simulink model "espesadorReal_1202"  (R2017a)
settings: Solver=VariableStepAuto  StartTime=0.0  StopTime=simTime  RelTol=1e-3  EnableMultiTasking=on
values from neighbouring files (symbols this model uses):
  a1 = 29.6547    [parametrosEmpty.m]
  a2 = 1.8198    [parametrosEmpty.m]
  a3 = 13.2250    (= 13.225)    [parametrosEmpty.m]
  B = 12    [parametrosEmpty.m]
  b0 = -1.3102    [parametrosEmpty.m]
  b1 = 25.8137    [parametrosEmpty.m]
  b2 = 40.3845    [parametrosEmpty.m]
  b3 = 78.1795    [parametrosEmpty.m]
  b4 = 1000    [parametrosEmpty.m]
  c0 = 1.6005e+03    (= 1600.5)    [parametrosEmpty.m]
  c1 = -512.8365    [parametrosEmpty.m]
  Cdata = linspace(0,phi_max,M)    [parametrosEmpty.m]
  Ddata = zeros(size(Cdata))    [parametrosEmpty.m]
  Dt = 1    [parametrosEmpty.m]
  Dz = (B+H)/N    (= 0.0690476190476)    [parametrosEmpty.m]
  jf = ceil(H/Dz)    [parametrosEmpty.m]
  kappa = 220.97    [parametrosEmpty.m]
  L = zeros(2,N+3)    [parametrosEmpty.m]
  lambda = 1./(Dz*A)    [parametrosEmpty.m]
  m = 8.68    [parametrosEmpty.m]
  mu = lambda/Dz    [parametrosEmpty.m]
  N = 210    [parametrosEmpty.m]
  n_rz = 9.65    [parametrosEmpty.m]
  phi0 = zeros(N+3,1)    [parametrosEmpty.m]
  phi_c = 0.2    [parametrosEmpty.m]
  phi_f = weight_to_volume_fraction(0.1,rho_s,rho_f)    [parametrosEmpty.m]
  rho_f = 1000    [parametrosEmpty.m]
  rho_s = 2750    [parametrosEmpty.m]
  theta = 0.2    [parametrosEmpty.m]
  u10 = zeros(N+3,1)    [parametrosEmpty.m]
  u20 = zeros(N+3,1)    [parametrosEmpty.m]
  u30 = zeros(N+3,1)    [parametrosEmpty.m]
  v_max = 25/3600    (= 0.00694444444444)    [parametrosEmpty.m]
  w0 = zeros(N+3,1)    [parametrosEmpty.m]
  y = abs(filter(b,1,SimResults.DV(dv).TimeSeries))    [plotter.m]
  Z = (-(H+Dz):Dz:(B+Dz))'    [parametrosEmpty.m]
undefined symbols (not defined in the file or in its folder): A, Cf_seed, Cf_sigma, Cz, DiscIntNeverNeededParam, p1_seed, p1_sigma, Qf_seed, Qf_sigma, startThickener
settings Model: SimulationMode=rapid-accelerator  ExtModeTrigDuration=100  Creator=pablo  LastModifiedBy=Pablo Diaz
settings DataIOCC: SaveOutput=off  StateSaveName=tmp_raccel_xout  SignalLoggingName=tmp_raccel_logsout
settings OptimizationCC: EfficientMapNaN2IntZero=off  LifeSpan=inf
settings DebuggingCC: SFUnexpectedBacktrackingDiag=warning  SFNoUnconditionalDefaultTransitionDiag=warning  SFExecutionAtInitializationDiag=none
settings HardwareCC: TargetBitPerPointer=64  TargetBitPerSizeT=64  TargetBitPerPtrDiffT=64  TargetLongLongMode=on  TargetIntDivRoundTo=Zero  TargetEndianess=LittleEndian  TargetWordSize=64  TargetHWDeviceType=MATLAB Host  ProdEqTarget=off
settings RTWCC: SystemTargetFile=raccel.tlc  TemplateMakefile=raccel_default_tmf  RTWVerbose=off  RTWUseSimCustomCode=on
settings CodeAppCC: GenerateComments=off  MaxIdLength=128  MangleLength=10  SimulinkBlockComments=off
settings RaccelTargetCC: GeneratePreprocessorConditionals=Use local settings  ERTFirstTimeCompliant=off  MultiInstanceERTCode=off  ENABLE_SLEXEC_SSBRIDGE=0  RTWCAPIParams=on
settings ConfigComp: CovMetricSettings=dw  CovHtmlReporting=on  CovSaveCumulativeToWorkspaceVar=on  CovSaveSingleToWorkspaceVar=on  CovExternalEMLEnable=off

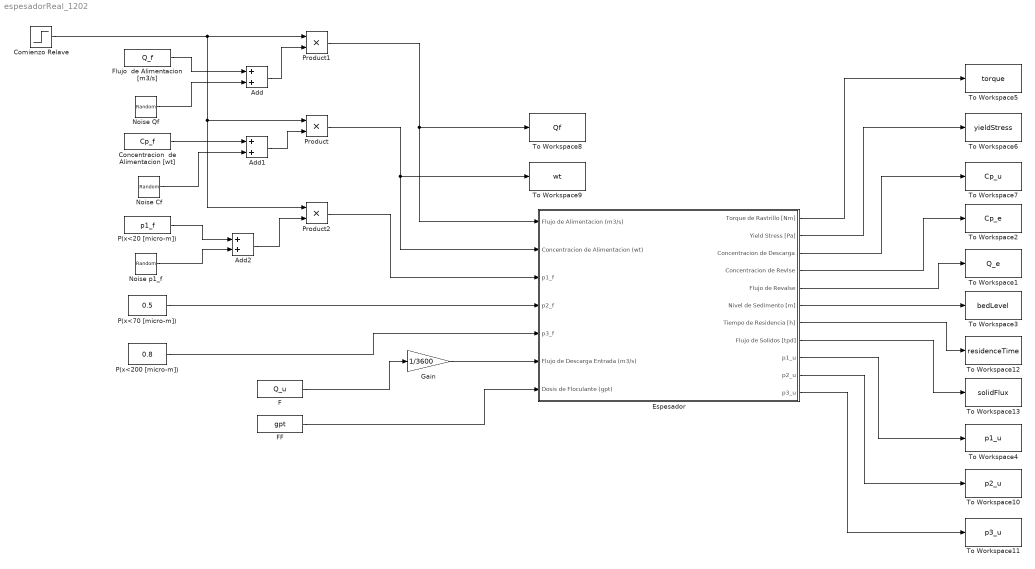
== system espesadorReal_1202 ==
  Add : Sum
  Add1 : Sum
  Add2 : Sum
  Comienzo Relave : Step  Time=startThickener  SampleTime=0
  Concentracion  de Alimentacion [wt] : FromWorkspace  VariableName=Cp_f  SampleTime=0
  Espesador : Subsystem
  F : FromWorkspace  VariableName=Q_u  SampleTime=0
  FF : FromWorkspace  VariableName=gpt  SampleTime=0
  Flujo  de Alimentacion [m3/s] : FromWorkspace  VariableName=Q_f  SampleTime=0
  Gain : Gain  Gain=1/3600
  Noise Cf : RandomNumber  Variance=Cf_sigma^2  Seed=Cf_seed  SampleTime=30*Dt
  Noise Qf : RandomNumber  Variance=Qf_sigma^2  Seed=Qf_seed  SampleTime=30*Dt
  Noise p1_f : RandomNumber  Variance=p1_sigma^2  Seed=p1_seed  SampleTime=30*Dt
  P(x<20 [micro-m]) : FromWorkspace  VariableName=p1_f  SampleTime=0
  P(x<200 [micro-m]) : Constant  Value=0.8
  P(x<70 [micro-m]) : Constant  Value=0.5
  Product : Product
  Product1 : Product
  Product2 : Product
  To Workspace1 : ToWorkspace  VariableName=Q_e  SaveFormat=Structure With Time  SampleTime=-1
  To Workspace10 : ToWorkspace  VariableName=p2_u  SaveFormat=Structure With Time  SampleTime=-1
  To Workspace11 : ToWorkspace  VariableName=p3_u  SaveFormat=Structure With Time  SampleTime=-1
  To Workspace12 : ToWorkspace  VariableName=residenceTime  SaveFormat=Structure With Time  SampleTime=-1
  To Workspace13 : ToWorkspace  VariableName=solidFlux  SaveFormat=Structure With Time  SampleTime=-1
  To Workspace2 : ToWorkspace  VariableName=Cp_e  SaveFormat=Structure With Time  SampleTime=-1
  To Workspace3 : ToWorkspace  VariableName=bedLevel  SaveFormat=Structure With Time  SampleTime=-1
  To Workspace4 : ToWorkspace  VariableName=p1_u  SaveFormat=Structure With Time  SampleTime=-1
  To Workspace5 : ToWorkspace  VariableName=torque  SaveFormat=Structure With Time  SampleTime=-1
  To Workspace6 : ToWorkspace  VariableName=yieldStress  SaveFormat=Structure With Time  SampleTime=-1
  To Workspace7 : ToWorkspace  VariableName=Cp_u  SaveFormat=Structure With Time  SampleTime=-1
  To Workspace8 : ToWorkspace  VariableName=Qf  SaveFormat=Structure With Time  SampleTime=-1
  To Workspace9 : ToWorkspace  VariableName=wt  SaveFormat=Structure With Time  SampleTime=-1
  wires:
  Espesador/1(Torque de Rastrillo [Nm]) -> To Workspace5/1
  Espesador/2(Yield Stress [Pa]) -> To Workspace6/1
  Espesador/3(Concentracion de Descarga) -> To Workspace7/1
  Espesador/4(Concentracion de Revlse) -> To Workspace2/1
  Espesador/5(Flujo de Revalse) -> To Workspace1/1
  Espesador/6(Nivel de Sedimento [m]) -> To Workspace3/1
  Espesador/9("p1_u ") -> To Workspace4/1
  Espesador/10("p2_u ") -> To Workspace10/1
  Espesador/11(p3_u) -> To Workspace11/1
  P(x<200 [micro-m])/1 -> Espesador/5(p3_f)
  Product2/1 -> Espesador/3(p1_f)
  P(x<70 [micro-m])/1 -> Espesador/4(p2_f)
  Product/1 -> Espesador/2(Concentracion de Alimentacion (wt)), To Workspace9/1
  Comienzo Relave/1 -> Product2/1, Product/1, Product1/1
  Flujo  de Alimentacion [m3/s]/1 -> Add/1
  Product1/1 -> Espesador/1(Flujo de Alimentacion (m3/s)), To Workspace8/1
  F/1 -> Gain/1
  FF/1 -> Espesador/7(Dosis de Floculante (gpt))
  Noise Qf/1 -> Add/2
  Add/1 -> Product1/2
  Concentracion  de Alimentacion [wt]/1 -> Add1/1
  Noise Cf/1 -> Add1/2
  Add1/1 -> Product/2
  Add2/1 -> Product2/2
  P(x<20 [micro-m])/1 -> Add2/1
  Noise p1_f/1 -> Add2/2
  Espesador/7(Tiempo de Residencia [h]) -> To Workspace12/1
  Espesador/8(Flujo de Solidos [tpd]) -> To Workspace13/1
  Gain/1 -> Espesador/6(Flujo de Descarga Entrada (m3/s))

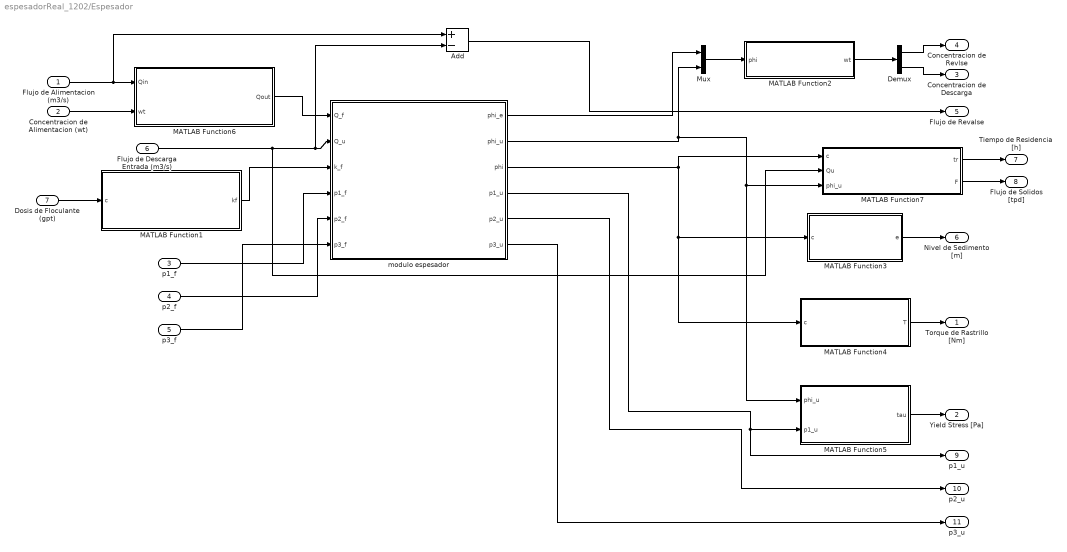
== system espesadorReal_1202/Espesador ==
  Flujo de Alimentacion (m3/s) : Inport
  Concentracion de Alimentacion (wt) : Inport  Port=2
  p1_f : Inport  Port=3
  p2_f : Inport  Port=4
  p3_f : Inport  Port=5
  Flujo de Descarga Entrada (m3/s) : Inport  Port=6
  Dosis de Floculante (gpt) : Inport  Port=7
  Add : Sum  Inputs=+-
  Demux : Demux  Outputs=2
  MATLAB Function1 : MATLAB Function  TreatAsAtomicUnit=on
  MATLAB Function2 : MATLAB Function  TreatAsAtomicUnit=on
  MATLAB Function3 : MATLAB Function  TreatAsAtomicUnit=on
  MATLAB Function4 : MATLAB Function  TreatAsAtomicUnit=on
  MATLAB Function5 : MATLAB Function  TreatAsAtomicUnit=on
  MATLAB Function6 : MATLAB Function  TreatAsAtomicUnit=on
  MATLAB Function7 : MATLAB Function  TreatAsAtomicUnit=on
  Mux : Mux  Inputs=2
  modulo espesador : Subsystem
  Torque de Rastrillo [Nm] : Outport
  Yield Stress [Pa] : Outport  Port=2
  Concentracion de Descarga : Outport  Port=3
  Concentracion de Revlse : Outport  Port=4
  Flujo de Revalse : Outport  Port=5
  Nivel de Sedimento [m] : Outport  Port=6
  Tiempo de Residencia [h] : Outport  Port=7
  Flujo de Solidos [tpd] : Outport  Port=8
  "p1_u " : Outport  Port=9
  "p2_u " : Outport  Port=10
  p3_u : Outport  Port=11
  wires:
  MATLAB Function3/1(e) -> Nivel de Sedimento [m]/1
  MATLAB Function4/1(T) -> Torque de Rastrillo [Nm]/1
  MATLAB Function5/1(tau) -> Yield Stress [Pa]/1
  Dosis de Floculante (gpt)/1 -> MATLAB Function1/1(c)
  Flujo de Descarga Entrada (m3/s)/1 -> MATLAB Function7/2(Qu), Add/2, modulo espesador/2(Q_u)
  MATLAB Function1/1(kf) -> modulo espesador/3(k_f)
  modulo espesador/1(phi_e) -> Mux/1
  modulo espesador/2(phi_u) -> MATLAB Function7/3(phi_u), MATLAB Function5/1(phi_u), Mux/2
  modulo espesador/5(p2_u) -> "p2_u "/1
  modulo espesador/3(phi) -> MATLAB Function7/1(c), MATLAB Function3/1(c), MATLAB Function4/1(c)
  p1_f/1 -> modulo espesador/4(p1_f)
  p2_f/1 -> modulo espesador/5("p2_f ")
  modulo espesador/4(p1_u) -> "p1_u "/1, MATLAB Function5/2(p1_u)
  Mux/1 -> MATLAB Function2/1(phi)
  MATLAB Function2/1(wt) -> Demux/1
  Demux/1 -> Concentracion de Revlse/1
  Demux/2 -> Concentracion de Descarga/1
  p3_f/1 -> modulo espesador/6(p3_f)
  modulo espesador/6(p3_u) -> p3_u/1
  MATLAB Function6/1(Qout) -> modulo espesador/1(Q_f)
  Flujo de Alimentacion (m3/s)/1 -> Add/1, MATLAB Function6/1(Qin)
  Concentracion de Alimentacion (wt)/1 -> MATLAB Function6/2(wt)
  MATLAB Function7/1(tr) -> Tiempo de Residencia [h]/1
  MATLAB Function7/2(F) -> Flujo de Solidos [tpd]/1
  Add/1 -> Flujo de Revalse/1

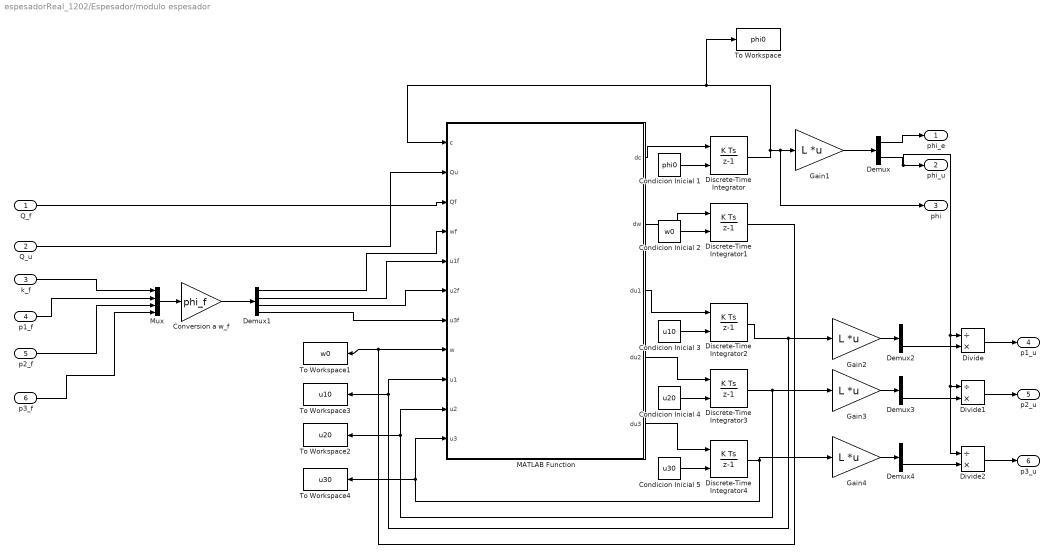
== system espesadorReal_1202/Espesador/modulo espesador ==
  Q_f : Inport
  Q_u : Inport  Port=2
  k_f : Inport  Port=3
  p1_f : Inport  Port=4
  "p2_f " : Inport  Port=5
  p3_f : Inport  Port=6
  Condicion Inicial 1 : Constant  Value=phi0
  Condicion Inicial 2 : Constant  Value=w0
  Condicion Inicial 3 : Constant  Value=u10
  Condicion Inicial 4 : Constant  Value=u20
  Condicion Inicial 5 : Constant  Value=u30
  Conversion a w_f : Gain  Gain=phi_f
  Demux{,2..4} (4 alike) : Demux  Outputs=2
  Demux1 : Demux
  Discrete-Time Integrator{,1..4} (5 alike) : DiscreteIntegrator  InitialConditionSource=external  InitialConditionSetting=State (most efficient)  SampleTime=Dt  ICPrevOutput=DiscIntNeverNeededParam  ICPrevScaledInput=DiscIntNeverNeededParam
  Divide : Product  Inputs=/*
  Divide1 : Product  Inputs=/*
  Divide2 : Product  Inputs=/*
  Gain{1..4} (4 alike) : Gain  Gain=L  Multiplication=Matrix(K*u) (u vector)
  MATLAB Function : MATLAB Function  TreatAsAtomicUnit=on
  Mux : Mux
  To Workspace : ToWorkspace  VariableName=phi0  SampleTime=-1
      settings: MaxDataPoints=1
  To Workspace1 : ToWorkspace  VariableName=w0  SampleTime=-1
      settings: MaxDataPoints=1
  To Workspace2 : ToWorkspace  VariableName=u20  SampleTime=-1
      settings: MaxDataPoints=1
  To Workspace3 : ToWorkspace  VariableName=u10  SampleTime=-1
      settings: MaxDataPoints=1
  To Workspace4 : ToWorkspace  VariableName=u30  SampleTime=-1
      settings: MaxDataPoints=1
  phi_e : Outport
  phi_u : Outport  Port=2
  phi : Outport  Port=3
  p1_u : Outport  Port=4
  p2_u : Outport  Port=5
  p3_u : Outport  Port=6
  wires:
  Discrete-Time Integrator/1 -> MATLAB Function/1(c), To Workspace/1, phi/1, Gain1/1
  Gain1/1 -> Demux/1
  Demux/1 -> phi_e/1
  Demux/2 -> Divide2/1, Divide1/1, Divide/1, phi_u/1
  MATLAB Function/1(dc) -> Discrete-Time Integrator/1
  Condicion Inicial 1/1 -> Discrete-Time Integrator/2
  Condicion Inicial 2/1 -> Discrete-Time Integrator1/2
  MATLAB Function/2(dw) -> Discrete-Time Integrator1/1
  Discrete-Time Integrator1/1 -> MATLAB Function/8(w), To Workspace1/1
  Q_f/1 -> MATLAB Function/3(Qf)
  Q_u/1 -> MATLAB Function/2(Qu)
  "p2_f "/1 -> Mux/3
  Mux/1 -> Conversion a w_f/1
  Conversion a w_f/1 -> Demux1/1
  Demux1/1 -> MATLAB Function/4(wf)
  Demux1/2 -> MATLAB Function/5(u1f)
  Demux1/3 -> MATLAB Function/6(u2f)
  Demux1/4 -> MATLAB Function/7(u3f)
  p3_f/1 -> Mux/4
  p1_f/1 -> Mux/2
  k_f/1 -> Mux/1
  Condicion Inicial 5/1 -> Discrete-Time Integrator4/2
  Condicion Inicial 4/1 -> Discrete-Time Integrator3/2
  MATLAB Function/5(du3) -> Discrete-Time Integrator4/1
  Discrete-Time Integrator4/1 -> To Workspace4/1, MATLAB Function/11(u3), Gain4/1
  MATLAB Function/4(du2) -> Discrete-Time Integrator3/1
  Discrete-Time Integrator3/1 -> Gain3/1, To Workspace2/1, MATLAB Function/10(u2)
  Condicion Inicial 3/1 -> Discrete-Time Integrator2/2
  MATLAB Function/3(du1) -> Discrete-Time Integrator2/1
  Discrete-Time Integrator2/1 -> Gain2/1, MATLAB Function/9(u1), To Workspace3/1
  Gain2/1 -> Demux2/1
  Demux2/2 -> Divide/2
  Divide/1 -> p1_u/1
  Gain3/1 -> Demux3/1
  Gain4/1 -> Demux4/1
  Divide1/1 -> p2_u/1
  Divide2/1 -> p3_u/1
  Demux3/2 -> Divide1/2
  Demux4/2 -> Divide2/2

== matlab function espesadorReal_1202/Espesador/MATLAB Function1 ==
  data: c input size=1; b0 parameter size=1; b1 parameter; kf output size=1; b2 parameter; b3 parameter; b4 parameter; v_max parameter
function kf = modelo_floculacion(c, b0, b1, b2, b3, b4, v_max)%#codegen

v = (b0+b1*(b2-c).*exp(-(c-b3).^2/b4))/3600;
kf = v/v_max;

== matlab function espesadorReal_1202/Espesador/modulo espesador/MATLAB Function ==
  data: c input size=N+3; Qu input size=1; Qf input size=1; wf input size=1; dc output size=N+3 [0..1]; dw output size=N+3; v_max parameter; n_rz parameter; lambda parameter; mu parameter; y parameter; jf parameter; N parameter; Dt parameter; Cdata parameter; Ddata parameter; phi_f parameter size=1; u1f input; u2f input; u3f input; w input size=N+3 [0..1]; du1 output; du2 output; du3 output; u1 input size=N+3; u2 input size=N+3; u3 input size=N+3
function [ dc, dw, du1, du2, du3] = modelo_espesador( c, Qu, Qf, wf, v_max, n_rz, lambda, mu, y, jf, N, Dt, Cdata, Ddata, phi_f, u1f, u2f, u3f, w, u1, u2, u3)%#codegen
%Metodo Numerico:
% "Modeling and controlling clarifier-thickeners fed by suspensions with
% time dependant properties" - Betancourt et al. 2014

%Variables Entrada:
% c = solid volume fraction j=-1...N+1
% w = conserved quantity j=-1...N+1
% cf = feed solid volume fraction (scalar)
% wf = feed value of conserved quantity (scalar)
% Qf = feed volume flow (m3/s)
% Qu = under-flow volume flow (m3/s)

%Variables de Salida:
% c = solid volume fraction j=-1...N+1
% w = conserved quantity j=-1...N+1
% Qe = effluent-flow volume flow (m3/s)
% cu = solid volume fraction of under-flow
% ce = solid volume fraction of effluent-flow

Qe = Qf - Qu;

assert (N < 1000);
assert (jf < 1000);

q = zeros(N+4,1);
dc1 = zeros(N+3,1);
dw1 = zeros(N+3,1);
du11 = zeros(N+3,1);
du21 = zeros(N+3,1);
du31 = zeros(N+3,1);
q(1:jf+2) = -Qe;
q(jf+3:end) = Qu;

%First step: linear contributions of the flux
dc1(1:jf+1) = - lambda(1:jf+1).*(q(2:jf+2).*(c(2:jf+2)-phi_f)-q(1:jf+1).*(c(1:jf+1)-phi_f));
dc1(jf+2) = - lambda(jf+2).*(q(jf+3).*(c(jf+2)-phi_f)-q(jf+2).*(c(jf+2)-phi_f));
dc1(jf+3:end) = - lambda(jf+3:end).*(q(jf+4:end).*(c(jf+3:end)-phi_f)-q(jf+3:end-1).*(c(jf+2:end-1)-phi_f));

c1 = c + Dt*dc1;

D = numerical_compression_flux(c1,Ddata,Cdata);
Dp = [D(2:end); 0]; Dm = [0; D(1:end-1)];

dw1(1:jf+1) = - lambda(1:jf+1).*(q(2:jf+2).*(w(2:jf+2)-wf)-q(1:jf+1).*(w(1:jf+1)-wf));
dw1(jf+2) = - lambda(jf+2).*(q(jf+3).*(w(jf+2)-wf)-q(jf+2).*(w(jf+2)-wf));
dw1(jf+3:end) = - lambda(jf+3:end).*(q(jf+4:end).*(w(jf+3:end)-wf)-q(jf+3:end-1).*(w(jf+2:end-1)-wf));

w1 = w + Dt*dw1;

du11(1:jf+1) = - lambda(1:jf+1).*(q(2:jf+2).*(u1(2:jf+2)-u1f)-q(1:jf+1).*(u1(1:jf+1)-u1f));
du11(jf+2) = - lambda(jf+2).*(q(jf+3).*(u1(jf+2)-u1f)-q(jf+2).*(u1(jf+2)-u1f));
du11(jf+3:end) = - lambda(jf+3:end).*(q(jf+4:end).*(u1(jf+3:end)-u1f)-q(jf+3:end-1).*(u1(jf+2:end-1)-u1f));

u11 = u1 + Dt*du11;

du21(1:jf+1) = - lambda(1:jf+1).*(q(2:jf+2).*(u2(2:jf+2)-u2f)-q(1:jf+1).*(u2(1:jf+1)-u2f));
du21(jf+2) = - lambda(jf+2).*(q(jf+3).*(u2(jf+2)-u2f)-q(jf+2).*(u2(jf+2)-u2f));
du21(jf+3:end) = - lambda(jf+3:end).*(q(jf+4:end).*(u2(jf+3:end)-u2f)-q(jf+3:end-1).*(u2(jf+2:end-1)-u2f));

u21 = u2 + Dt*du21;

du31(1:jf+1) = - lambda(1:jf+1).*(q(2:jf+2).*(u3(2:jf+2)-u3f)-q(1:jf+1).*(u3(1:jf+1)-u3f));
du31(jf+2) = - lambda(jf+2).*(q(jf+3).*(u3(jf+2)-u3f)-q(jf+2).*(u3(jf+2)-u3f));
du31(jf+3:end) = - lambda(jf+3:end).*(q(jf+4:end).*(u3(jf+3:end)-u3f)-q(jf+3:end-1).*(u3(jf+2:end-1)-u3f));

u31 = u3 + Dt*du31;

%Variable computation
k=c1; k(c1>eps)=w1(c1>eps)./c1(c1>eps);

V=y(3:N+2).*k(3:N+2).*v_hs(c1(3:N+2),v_max,n_rz); Vp = [0; V; 0; 0]; Vm = [0; 0; V; 0];

k1 = (c1(2:N+1)>=c1(3:N+2)).*k(2:N+1) + (c1(2:N+1)<c1(3:N+2)).*k(3:N+2); k1p = [0; k1; 0; 0]; k1m = [0; 0; k1; 0];

w2 = (c1(2:N+1)>=c1(3:N+2)).*w1(2:N+1) + (c1(2:N+1)<c1(3:N+2)).*w1(3:N+2); w2p = [0; w2; 0; 0]; w2m = [0; 0; w2; 0];

u12 = (c1(2:N+1)>=c1(3:N+2)).*u11(2:N+1) + (c1(2:N+1)<c1(3:N+2)).*u11(3:N+2); u12p = [0; u12; 0; 0]; u12m = [0; 0; u12; 0];

u22 = (c1(2:N+1)>=c1(3:N+2)).*u21(2:N+1) + (c1(2:N+1)<c1(3:N+2)).*u21(3:N+2); u22p = [0; u22; 0; 0]; u22m = [0; 0; u22; 0];

u32 = (c1(2:N+1)>=c1(3:N+2)).*u31(2:N+1) + (c1(2:N+1)<c1(3:N+2)).*u31(3:N+2); u32p = [0; u32; 0; 0]; u32m = [0; 0; u32; 0];

yp = y(2:N+4); ym = y(1:N+3);

c1m = [0; c1(1:end-1)];
w1m = [0; w1(1:end-1)];
u11m = [0; u11(1:end-1)];
u21m = [0; u21(1:end-1)];
u31m = [0; u31(1:end-1)];

%Second step: non-linear contributions of the flux

dc = dc1 - lambda.*(Vp.*c1-Vm.*c1m) + mu.*(yp.*w2p.*(Dp-D)-ym.*w2m.*(D-Dm));
dw = dw1 - lambda.*(Vp.*w1-Vm.*w1m) + mu.*(yp.*w2p.*k1p.*(Dp-D)-ym.*w2m.*k1m.*(D-Dm));
du1 = du11 - lambda.*(Vp.*u11-Vm.*u11m) + mu.*(yp.*u12p.*k1p.*(Dp-D)-ym.*u12m.*k1m.*(D-Dm));
du2 = du21 - lambda.*(Vp.*u21-Vm.*u21m) + mu.*(yp.*u22p.*k1p.*(Dp-D)-ym.*u22m.*k1m.*(D-Dm));
du3 = du31 - lambda.*(Vp.*u31-Vm.*u31m) + mu.*(yp.*u32p.*k1p.*(Dp-D)-ym.*u32m.*k1m.*(D-Dm));

== matlab function espesadorReal_1202/Espesador/MATLAB Function2 ==
  data: phi input; wt output; rho_s parameter; rho_f parameter
function wt = volume_to_weight_fraction(phi, rho_s, rho_f)
%#codegen

wt = phi*rho_s./(phi*rho_s+(1-phi)*rho_f);

== matlab function espesadorReal_1202/Espesador/MATLAB Function3 ==
  data: c input; e output; phi_c parameter; Z parameter size=N+3; B parameter
function e = modelo_nivel_sedimento(c, phi_c, Z, B)%#codegen

if (sum(c>=phi_c)>=2)
    % If two or more layers exhibit concentration greater than phi_c, then
    % there is a sedimentation layer.
    e = min(Z(c>=phi_c));
    % The height of the sedimentation layer is measured from feedwell (z =
    % 0) to bottom (z = 12). The above command returns the minimum of the Z
    % that has a phi >= phi_c. Therefore, it returns the height measured
    % from the feedwell to the critical interphase. Therefore, it measures
    % the width of the interphase region.
    % The thickness of the sedimentation layer (from the bottom of the
    % thickener) is B-e.
else
    e = B;
end

== matlab function espesadorReal_1202/Espesador/MATLAB Function4 ==
  data: c input; T output; Cz parameter; a1 parameter; a2 parameter; a3 parameter
function T = modelo_torque_rastrillo(c,Cz,a1,a2,a3)
%#codegen

T = a1*(Cz'*c).^a2+a3;

== matlab function espesadorReal_1202/Espesador/MATLAB Function5 ==
  data: phi_u input; p1_u input; tau output; kappa parameter; m parameter; rho_s parameter; c0 parameter; c1 parameter; theta parameter; rho_f parameter
function tau = modelo_yield_stress(phi_u,p1_u,kappa,m,rho_s, c0,c1,theta, rho_f)
%#codegen

    rho = c0 + c1*(p1_u-theta).^2;
    wt = phi_u*rho_s./(phi_u*rho_s+(1-phi_u)*rho_f);
    Sr = rho.*rho_s./(rho_s-rho).*(1-wt)*1e-3;
    tau = kappa*Sr.^(-m);

== matlab function espesadorReal_1202/Espesador/MATLAB Function6 ==
  data: Qin input size=1; phi_f parameter; Qout output size=1; wt input size=1; rho_f parameter; rho_s parameter
function Qout = modelo_dilucion(Qin,phi_f, wt,rho_f, rho_s)%#codegen

phi = (wt*rho_f)/(wt*rho_f+(1-wt)*rho_s);

Qout = Qin*phi/phi_f;

== matlab function espesadorReal_1202/Espesador/MATLAB Function7 ==
  data: c input size=N+3; tr output; A parameter size=N+3; Dz parameter; F output; rho_s parameter; Qu input; phi_u input
function [tr, F] = modelo_tiempo_de_residencia(c, A, Dz, rho_s, Qu, phi_u)%#codegen

F = Qu*phi_u; %m3/s de solido
tr = (A'*c)*Dz/F/3600; %h
F = F*rho_s*3.6*24; %tpd de solido

end
